simulink model "Two_Wheel_sys"  (R2021b)
settings: Solver=VariableStepAuto  StartTime=0.0  StopTime=10.0  RelTol=1e-3
settings Model: Creator=Lorenzo  LastModifiedBy=Lorenzo

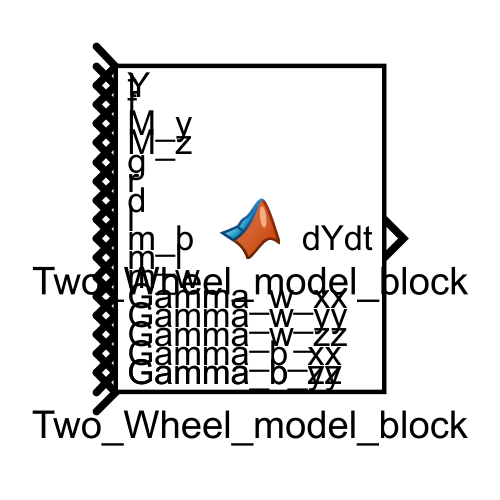
[thumbnail: Simulink's stored preview of the top-level diagram]
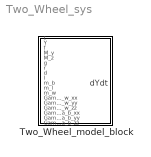
== system Two_Wheel_sys ==
  Two_Wheel_model_block : MATLAB Function  TreatAsAtomicUnit=on

== matlab function Two_Wheel_sys/Two_Wheel_model_block ==
  data: t input; dYdt output; Y input; f input; M_y input; M_z input; g input; r input; d input; l input; m_b input; m_l input; m_w input; Gamma_w_xx input; Gamma_w_yy input; Gamma_w_zz input; Gamma_b_xx input; Gamma_b_yy input; Gamma_b_zz input
function dYdt = Two_Wheel_model_block(t,Y,f,M_y,M_z,g,r,d,l,m_b,m_l,m_w,Gamma_w_xx,Gamma_w_yy,Gamma_w_zz,Gamma_b_xx,Gamma_b_yy,Gamma_b_zz)
%#codegen

%    This function was generated by the Symbolic Math Toolbox version 9.0.
%    15-Jul-2022 17:19:22

t2 = Y(1);
t3 = d.^2;
t4 = l.^2;
t5 = m_w.^2;
t6 = r.^2;
t7 = Gamma_b_yy.*Gamma_w_yy;
t8 = sin(t2);
t9 = Gamma_w_yy.*m_w.*t4;
t10 = Gamma_b_yy.*m_w.*t6.*3.0;
t11 = t4.*t5.*t6.*2.0;
t12 = t7+t9+t10+t11;
t13 = 1.0./t12;
dYdt = [Y(2);-t13.*(-Gamma_w_yy.*M_y-M_y.*m_w.*t6.*3.0+f.*l.*m_w.*t6+Gamma_w_yy.*g.*l.*t8+g.*l.*m_w.*t6.*t8.*3.0);Y(4);t6.*t13.*(Gamma_b_yy.*f-M_y.*l.*m_w+f.*m_w.*t4+g.*m_w.*t4.*t8);Y(6);(M_z.*t6.*2.0)./(Gamma_b_zz.*t6.*2.0+Gamma_w_yy.*t3+Gamma_w_zz.*t6.*4.0+m_w.*t3.*t6)];
